simulink model "Part3_2"  (R2022a)
settings: Solver=VariableStepAuto  StartTime=0.0  StopTime=1000  RelTol=1e-3
values from neighbouring files (symbols this model uses):
  D = diag([0.01, 0.01, 0.01])    [Driver33_NL.m]    (also in Driver_3.m; Driver_33.m; Driver_3NL.m)
  g = [0,0,-9.81]    [Driver33_NL.m]    (also in Driver_3.m; Driver_33.m; Driver_3NL.m)
  g2 = [0,0,0,-9.81]    [Driver33_NL.m]    (also in Driver_3.m; Driver_33.m; Driver_3NL.m)
  I = diag([3e-6, 3e-6, 1e-5])    [Driver33_NL.m]    (also in Driver_3.m; Driver_33.m; Driver_3NL.m)
  I_tf = diag([3e-6, 3e-6, 1e-5, 1])    [Driver33_NL.m]    (also in Driver_3.m; Driver_33.m; Driver_3NL.m)
  In = inv(I)    [Driver33_NL.m]    (also in Driver_3.m; Driver_33.m; Driver_3NL.m)
  k = 0.01    [Driver33_NL.m]    (also in Driver_3.m; Driver_33.m; Driver_3NL.m)
  K_d = 2.5*(1/2.65)    (= 0.943396226415)    [Driver33_NL.m]    (also in Driver_3.m; Driver_33.m; Driver_3NL.m)
  K_i = 0.2*(1/2.65)    (= 0.0754716981132)    [Driver33_NL.m]    (also in Driver_3.m; Driver_33.m; Driver_3NL.m)
  K_p = 1.9    [Driver33_NL.m]    (also in Driver_3.m; Driver_33.m; Driver_3NL.m)
  m = 0.5    [Driver33_NL.m]    (also in Driver_3.m; Driver_33.m; Driver_3NL.m)
  mvec = [1 ... (first row only)    [Driver33_NL.m]    (also in Driver_3.m; Driver_33.m; Driver_3NL.m)
  TF2 = inv(tf2)    [Driver33_NL.m]    (also in Driver_3.m; Driver_33.m; Driver_3NL.m)
  tf_34 = [L*k, 0, -L*k, 0 ... (first row only)    [Driver33_NL.m]    (also in Driver_3.m; Driver_33.m; Driver_3NL.m)
  u0 = [phi ... (first row only)    [Driver_3NL.m]
  u1 = [phi ... (first row only)    [Driver_3NL.m]
libraries: matrix_library x1
settings Model: Creator=askeo  LastModifiedBy=askeo

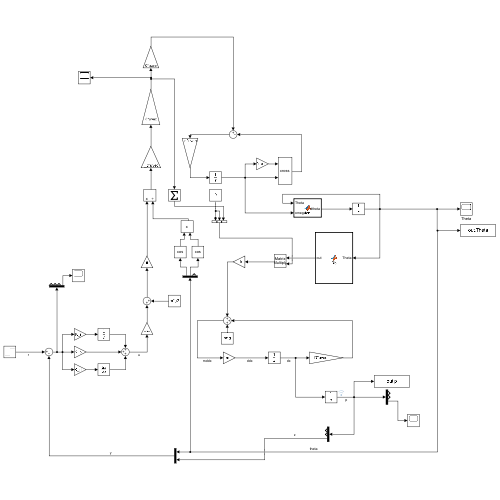
[thumbnail: Simulink's stored preview of the top-level diagram]
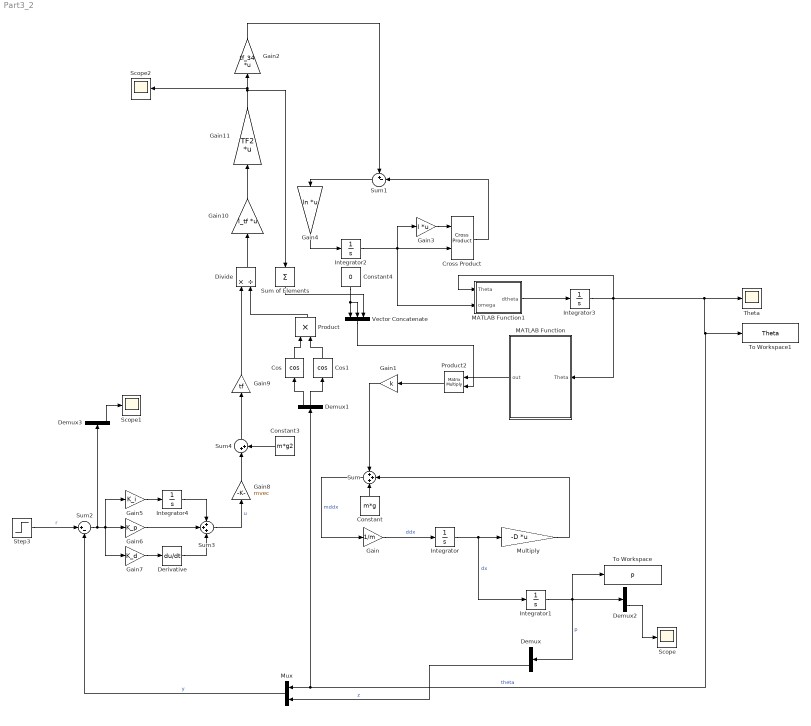
== system Part3_2 ==
  Constant : Constant  Value=m*g
  Constant3 : Constant  Value=m*g2
  Constant4 : Constant  Value=0
  Cos : Trigonometry  Operator=cos
  Cos1 : Trigonometry  Operator=cos
  Cross Product : matrix_library/Cross Product
      settings: SourceProductBaseCode=SL
  Demux : Demux  Outputs=3
  Demux1 : Demux  Outputs=3
  Demux2 : Demux  Outputs=3
  Demux3 : Demux
  Derivative : Derivative
  Divide : Product  Inputs=*/
  Gain : Gain  Gain=1/m
  Gain1 : Gain  Gain=k
  Gain10 : Gain  Gain=I_tf  Multiplication=Matrix(K*u) (u vector)
  Gain11 : Gain  Gain=TF2  Multiplication=Matrix(K*u) (u vector)
  Gain2 : Gain  Gain=tf_34  Multiplication=Matrix(K*u) (u vector)
  Gain3 : Gain  Gain=I  Multiplication=Matrix(K*u) (u vector)
  Gain4 : Gain  Gain=In  Multiplication=Matrix(K*u) (u vector)
  Gain5 : Gain  Gain=K_i
  Gain6 : Gain  Gain=K_p
  Gain7 : Gain  Gain=K_d
  Gain8 : Gain  Gain=mvec
  Gain9 : Gain  Gain=tf
  Integrator : Integrator  InitialCondition=[0;0;0]
  Integrator1 : Integrator  InitialCondition=[0;0;0]
  Integrator2 : Integrator  InitialCondition=[0;0;0]
  Integrator3 : Integrator  InitialCondition=[0; 0; 0]
  Integrator4 : Integrator
  MATLAB Function : MATLAB Function  TreatAsAtomicUnit=on
  MATLAB Function1 : MATLAB Function  TreatAsAtomicUnit=on
  Multiply : Gain  Gain=-D  Multiplication=Matrix(K*u) (u vector)
  Mux : Mux  Inputs=2
  Product : Product
  Product2 : Product  Multiplication=Matrix(*)
  Scope : Scope
  Scope1 : Scope
  Scope2 : Scope
  Step3 : Step  Time=500  Before=u0  After=u1  SampleTime=0
  Sum : Sum  Inputs=+++
  Sum of Elements : Sum  Inputs=+
  Sum1 : Sum  Inputs=+-|
  Sum2 : Sum  Inputs=|+-
  Sum3 : Sum  Inputs=+++
  Sum4 : Sum  Inputs=|++
  Theta : Scope
  To Workspace : ToWorkspace  VariableName=p  SampleTime=-1
  To Workspace1 : ToWorkspace  VariableName=Theta  SampleTime=0.001
  Vector Concatenate : Concatenate  NumInputs=3
  wires:
  Gain6/1 -> Sum3/2
  Sum4/1 -> Gain9/1
  Cos1/1 -> Product/2
  Gain5/1 -> Integrator4/1
  Product/1 -> Divide/2
  Gain8/1 -> Sum4/1
  Gain7/1 -> Derivative/1
  Constant3/1 -> Sum4/2
  Gain9/1 -> Divide/1
  Gain4/1 -> Integrator2/1
  Gain3/1 -> Cross Product/1
  Sum3/1 -> Gain8/1  "u"
  Constant/1 -> Sum/3
  Gain2/1 -> Sum1/1
  Sum1/1 -> Gain4/1
  Integrator4/1 -> Sum3/1
  Demux/3 -> Mux/2  "z"
  Integrator1/1 -> Demux2/1, Demux/1, To Workspace/1  "p"
  Integrator/1 -> Integrator1/1, Multiply/1  "dx"
  Gain1/1 -> Sum/1
  Multiply/1 -> Sum/2
  Cross Product/1 -> Sum1/2
  MATLAB Function1/1(dtheta) -> Integrator3/1
  Cos/1 -> Product/1
  Integrator3/1 -> MATLAB Function1/1(Theta), MATLAB Function/1(Theta), Mux/1, Demux1/1, To Workspace1/1, Theta/1  "theta"
  Integrator2/1 -> MATLAB Function1/2(omega), Gain3/1, Cross Product/2
  Product2/1 -> Gain1/1
  Sum/1 -> Gain/1  "mddx"
  Sum2/1 -> Gain6/1, Gain7/1, Gain5/1, Demux3/1
  Demux1/2 -> Cos1/1
  Mux/1 -> Sum2/2  "y"
  Demux1/1 -> Cos/1
  Gain/1 -> Integrator/1  "ddx"
  Derivative/1 -> Sum3/3
  Divide/1 -> Gain10/1
  Constant4/1 -> Vector Concatenate/2, Vector Concatenate/1
  Sum of Elements/1 -> Vector Concatenate/3
  Vector Concatenate/1 -> Product2/2
  Gain10/1 -> Gain11/1
  Gain11/1 -> Scope2/1, Gain2/1, Sum of Elements/1
  MATLAB Function/1(out) -> Product2/1
  Demux2/3 -> Scope/1
  Demux3/4 -> Scope1/1
  Step3/1 -> Sum2/1  "r"

== matlab function Part3_2/MATLAB Function1 ==
  data: dtheta output; Theta input; omega input
function dtheta = fcn(Theta, omega)

C = [1, 0, -sin(Theta(2))
    0, cos(Theta(1)), cos(Theta(2))*sin(Theta(1))
    0, -sin(Theta(1)), cos(Theta(2))*cos(Theta(1))];

dtheta = inv(C)*omega;
end

== matlab function Part3_2/MATLAB Function ==
  data: Theta input; out output
function out = Rb(Theta)

phi = Theta(1);
theta = Theta(2);
psi = Theta(3);

rbi = [cos(psi)*cos(theta), cos(psi)*sin(theta)*sin(phi) - sin(psi)*cos(phi), sin(psi)*sin(phi) + cos(psi)*sin(theta)*cos(phi)
    sin(psi)*cos(theta), cos(psi)*cos(phi) + sin(psi)*sin(theta)*sin(phi), sin(psi)*sin(theta)*sin(phi) - cos(psi)*sin(phi)
    -sin(theta), cos(theta)*sin(phi), cos(theta)*cos(phi)];

out = rbi;
end
